simulink model "vehiclelatdynamic"  (R2017a)
settings: Solver=VariableStepAuto  StartTime=0.0  StopTime=100  RelTol=1e-3
values from neighbouring files (symbols this model uses):
  A = [0,1,0,0 ... (first row only)    [control.m]
  B1 = [0; 2*C_f/m; 0; 2*C_f*lf/I_z]    [control.m]
  B2 = [0; -(2*C_f*lf - 2*C_r*lr)/(m*V_x)-V_x; 0; -(2*C_f*lf^2 + 2*C_r*lr^2)/(I_z*V_x)]    [control.m]
  delta_ff = (m * V_x^2)/(Radi*L)*( (lr)/(2*C_f) - (lf)/(2*C_r) + (lf)/(2*C_r)*K(3) ) + L/Radi - lr/Radi * K(3)    [control.m]
  K = lqr(A,B1,Q,R,0)    [control.m]
  phi_des_d = V_x/Radi    [road.m]
settings Model: Creator=liuheng  LastModifiedBy=liuheng

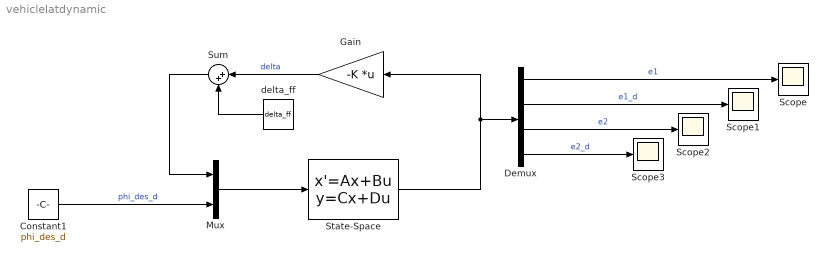
== system vehiclelatdynamic ==
  Constant1 : Constant  Value=phi_des_d
  Demux : Demux
  Gain : Gain  Gain=-K  Multiplication=Matrix(K*u)
  Mux : Mux  Inputs=2
  Scope{,1..3} (4 alike) : Scope
  State-Space : StateSpace  A=A  B=[B1,B2]  C=eye(4)  D=[0,0;0,0;0,0;0,0]  X0=[1;0;0;0]
  Sum : Sum  Inputs=|++
  delta_ff : Constant  Value=delta_ff
  wires:
  Mux/1 -> State-Space/1
  Constant1/1 -> Mux/2  "phi_des_d"
  State-Space/1 -> Gain/1, Demux/1
  Demux/1 -> Scope/1  "e1"
  Demux/2 -> Scope1/1  "e1_d"
  Demux/3 -> Scope2/1  "e2"
  Demux/4 -> Scope3/1  "e2_d"
  Gain/1 -> Sum/1  "delta"
  delta_ff/1 -> Sum/2
  Sum/1 -> Mux/1
